simulink library "inp"  (R2021b)
settings: Solver=VariableStepAuto  StartTime=0.0  StopTime=10.0  RelTol=1e-3
undefined symbols (not defined in the file): C_TASK_5MS_S, FALSE, KINP_AcoreReadyToSlp_flg_ovrdflg, KINP_AcoreReadyToSlp_flg_ovrdval, KINP_AllowMovThd_OTA_enum_ovrdflg, KINP_AllowMovThd_OTA_enum_ovrdval, KINP_APSAngleTarget_Deg_ovrdflg, KINP_APSAngleTarget_Deg_ovrdval, KINP_APSDecReq_mps2_ovrdflg, KINP_APSDecReq_mps2_ovrdval, KINP_APSDecReqA_flg_ovrdflg, KINP_APSDecReqA_flg_ovrdval, KINP_APSDFLL_cm_ovrdflg, KINP_APSDFLL_cm_ovrdval, KINP_APSDFLR_cm_ovrdflg, KINP_APSDFLR_cm_ovrdval, KINP_APSDRLL_cm_ovrdflg, KINP_APSDRLL_cm_ovrdval, KINP_APSDRLR_cm_ovrdflg, KINP_APSDRLR_cm_ovrdval, KINP_APSExitCondition_enum_ovrdflg, KINP_APSExitCondition_enum_ovrdval, KINP_APSHWVer_enum_ovrdflg, KINP_APSHWVer_enum_ovrdval, KINP_APSProgressPCT_pct_ovrdflg, KINP_APSProgressPCT_pct_ovrdval, KINP_APSPwrReq_enum_ovrdflg, KINP_APSPwrReq_enum_ovrdval, KINP_APSReq_enum_ovrdflg, KINP_APSReq_enum_ovrdval, KINP_APSRQDisplay_enum_ovrdflg, KINP_APSRQDisplay_enum_ovrdval, KINP_APSRqEPASCtrl_flg_ovrdflg, KINP_APSRqEPASCtrl_flg_ovrdval, KINP_APSShiftPosnReq_enum_ovrdval, KINP_APSShiftPosnReq_enum_ovrflg, KINP_APSSpeedCMD_kph_ovrdval, KINP_APSSpeedCMD_kph_ovrflg, KINP_APSStaSystem_enum_ovrdflg, KINP_APSStaSystem_enum_ovrdval, KINP_APSSWVer_enum_ovrdflg, KINP_APSSWVer_enum_ovrdval, KINP_APSVMCReqA_flg_ovrdval, KINP_APSVMCReqA_flg_ovrflg, KINP_APSVRqEPASCtrl_flg_ovrdflg, KINP_APSVRqEPASCtrl_flg_ovrdval, KINP_AuxBattVolmV_mV_ovrdflg, KINP_AuxBattVolmV_mV_ovrdval, KINP_BTConnectSta_enum_ovrdflg, KINP_BTConnectSta_enum_ovrdval, KINP_CAASSta_enum_ovrdflg, KINP_CAASSta_enum_ovrdval, KINP_CAASVMCReqA_flg_ovrdval, KINP_CAASVMCReqA_flg_ovrflg, KINP_CAN1BusOff_flg_ovrdflg, KINP_CAN1BusOff_flg_ovrdval, KINP_CAN2BusOff_flg_ovrdflg, KINP_CAN2BusOff_flg_ovrdval, KINP_CAN3BusOff_flg_ovrdflg, KINP_CAN3BusOff_flg_ovrdval ... (+222)
libraries: FVT_lib x1035, hcu_lib x1
(part 30 of 33)

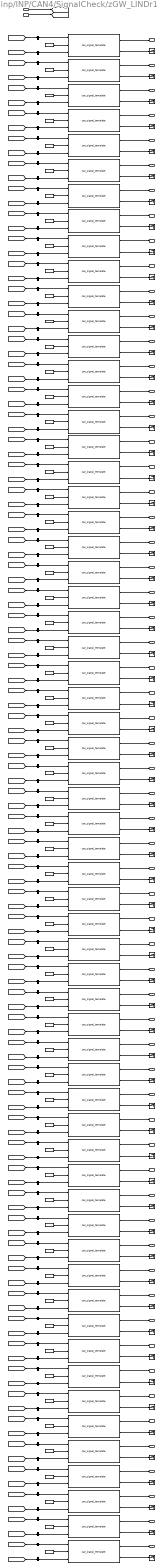
== system inp/INP/CAN4/SignalCheck/zGW_LINDr1 ==
  BHAL_outputs : Inport
  inp_CanValid_bus : Inport  Port=2
  CSWDimSw : FVT_lib/inp/can_signal_template  SystemSampleTime=-1  VariantActivationTime=update diagram  Latency=0  AutoFrameSizeCalculation=off
      link override defval: Value=KINP_CSWDimSw_flg_defval
      link override ovrdflg: Value=KINP_CSWDimSw_flg_ovrdflg
      link override ovrdval: Value=KINP_CSWDimSw_flg_ovrdval
  CSWFWasSwSta : FVT_lib/inp/can_signal_template  SystemSampleTime=-1  VariantActivationTime=update diagram  Latency=0  AutoFrameSizeCalculation=off
      link override defval: Value=KINP_CSWFWasSwSta_enum_defval
      link override ovrdflg: Value=KINP_CSWFWasSwSta_enum_ovrdflg
      link override ovrdval: Value=KINP_CSWFWasSwSta_enum_ovrdval
  CSWFWipSwSta : FVT_lib/inp/can_signal_template  SystemSampleTime=-1  VariantActivationTime=update diagram  Latency=0  AutoFrameSizeCalculation=off
      link override defval: Value=KINP_CSWFWipSwSta_enum_defval
      link override ovrdflg: Value=KINP_CSWFWipSwSta_enum_ovrdflg
      link override ovrdval: Value=KINP_CSWFWipSwSta_enum_ovrdval
  CSWPassSWSta : FVT_lib/inp/can_signal_template  SystemSampleTime=-1  VariantActivationTime=update diagram  Latency=0  AutoFrameSizeCalculation=off
      link override defval: Value=KINP_CSWPassSWSta_flg_defval
      link override ovrdflg: Value=KINP_CSWPassSWSta_flg_ovrdflg
      link override ovrdval: Value=KINP_CSWPassSWSta_flg_ovrdval
  CSWRWasSWSta : FVT_lib/inp/can_signal_template  SystemSampleTime=-1  VariantActivationTime=update diagram  Latency=0  AutoFrameSizeCalculation=off
      link override defval: Value=KINP_CSWRWasSWSta_enum_defval
      link override ovrdflg: Value=KINP_CSWRWasSWSta_enum_ovrdflg
      link override ovrdval: Value=KINP_CSWRWasSWSta_enum_ovrdval
  CSWRWipIntSwSta : FVT_lib/inp/can_signal_template  SystemSampleTime=-1  VariantActivationTime=update diagram  Latency=0  AutoFrameSizeCalculation=off
      link override defval: Value=KINP_CSWRWipIntSwSta_enum_defval
      link override ovrdflg: Value=KINP_CSWRWipIntSwSta_enum_ovrdflg
      link override ovrdval: Value=KINP_CSWRWipIntSwSta_enum_ovrdval
  CSWTurnSwSta : FVT_lib/inp/can_signal_template  SystemSampleTime=-1  VariantActivationTime=update diagram  Latency=0  AutoFrameSizeCalculation=off
      link override defval: Value=KINP_CSWTurnSwSta_enum_defval
      link override ovrdflg: Value=KINP_CSWTurnSwSta_enum_ovrdflg
      link override ovrdval: Value=KINP_CSWTurnSwSta_enum_ovrdval
  FAPWL01LINResponseError : FVT_lib/inp/can_signal_template  SystemSampleTime=-1  VariantActivationTime=update diagram  Latency=0  AutoFrameSizeCalculation=off
      link override defval: Value=KINP_FAPWL01LINResponseError_flg_defval
      link override ovrdflg: Value=KINP_FAPWL01LINResponseError_flg_ovrdflg
      link override ovrdval: Value=KINP_FAPWL01LINResponseError_flg_ovrdval
  LDrvMotorRelayError : FVT_lib/inp/can_signal_template  SystemSampleTime=-1  VariantActivationTime=update diagram  Latency=0  AutoFrameSizeCalculation=off
      link override defval: Value=KINP_LDrvMotorRelayError_flg_defval
      link override ovrdflg: Value=KINP_LDrvMotorRelayError_flg_ovrdflg
      link override ovrdval: Value=KINP_LDrvMotorRelayError_flg_ovrdval
  LDrvMotorRippleError : FVT_lib/inp/can_signal_template  SystemSampleTime=-1  VariantActivationTime=update diagram  Latency=0  AutoFrameSizeCalculation=off
      link override defval: Value=KINP_LDrvMotorRippleError_flg_defval
      link override ovrdflg: Value=KINP_LDrvMotorRippleError_flg_ovrdflg
      link override ovrdval: Value=KINP_LDrvMotorRippleError_flg_ovrdval
  LDrvValWdwOpened : FVT_lib/inp/can_signal_template  SystemSampleTime=-1  VariantActivationTime=update diagram  Latency=0  AutoFrameSizeCalculation=off
      link override defval: Value=KINP_LDrvValWdwOpened_pct_defval
      link override ovrdflg: Value=KINP_LDrvValWdwOpened_pct_ovrdflg
      link override ovrdval: Value=KINP_LDrvValWdwOpened_pct_ovrdval
  LDrvWdwPositionSts : FVT_lib/inp/can_signal_template  SystemSampleTime=-1  VariantActivationTime=update diagram  Latency=0  AutoFrameSizeCalculation=off
      link override defval: Value=KINP_LDrvWdwPositionSts_enum_defval
      link override ovrdflg: Value=KINP_LDrvWdwPositionSts_enum_ovrdflg
      link override ovrdval: Value=KINP_LDrvWdwPositionSts_enum_ovrdval
  LPasMotorRelayError : FVT_lib/inp/can_signal_template  SystemSampleTime=-1  VariantActivationTime=update diagram  Latency=0  AutoFrameSizeCalculation=off
      link override defval: Value=KINP_LPasMotorRelayError_flg_defval
      link override ovrdflg: Value=KINP_LPasMotorRelayError_flg_ovrdflg
      link override ovrdval: Value=KINP_LPasMotorRelayError_flg_ovrdval
  LPasMotorRippleError : FVT_lib/inp/can_signal_template  SystemSampleTime=-1  VariantActivationTime=update diagram  Latency=0  AutoFrameSizeCalculation=off
      link override defval: Value=KINP_LPasMotorRippleError_flg_defval
      link override ovrdflg: Value=KINP_LPasMotorRippleError_flg_ovrdflg
      link override ovrdval: Value=KINP_LPasMotorRippleError_flg_ovrdval
  LPasValWdwOpened : FVT_lib/inp/can_signal_template  SystemSampleTime=-1  VariantActivationTime=update diagram  Latency=0  AutoFrameSizeCalculation=off
      link override defval: Value=KINP_LPasValWdwOpened_pct_defval
      link override ovrdflg: Value=KINP_LPasValWdwOpened_pct_ovrdflg
      link override ovrdval: Value=KINP_LPasValWdwOpened_pct_ovrdval
  LPasWdwPositionSts : FVT_lib/inp/can_signal_template  SystemSampleTime=-1  VariantActivationTime=update diagram  Latency=0  AutoFrameSizeCalculation=off
      link override defval: Value=KINP_LPasWdwPositionSts_enum_defval
      link override ovrdflg: Value=KINP_LPasWdwPositionSts_enum_ovrdflg
      link override ovrdval: Value=KINP_LPasWdwPositionSts_enum_ovrdval
  LRLDMotorRelayError : FVT_lib/inp/can_signal_template  SystemSampleTime=-1  VariantActivationTime=update diagram  Latency=0  AutoFrameSizeCalculation=off
      link override defval: Value=KINP_LRLDMotorRelayError_flg_defval
      link override ovrdflg: Value=KINP_LRLDMotorRelayError_flg_ovrdflg
      link override ovrdval: Value=KINP_LRLDMotorRelayError_flg_ovrdval
  LRLDMotorRippleError : FVT_lib/inp/can_signal_template  SystemSampleTime=-1  VariantActivationTime=update diagram  Latency=0  AutoFrameSizeCalculation=off
      link override defval: Value=KINP_LRLDMotorRippleError_flg_defval
      link override ovrdflg: Value=KINP_LRLDMotorRippleError_flg_ovrdflg
      link override ovrdval: Value=KINP_LRLDMotorRippleError_flg_ovrdval
  LRLDValWdwOpened : FVT_lib/inp/can_signal_template  SystemSampleTime=-1  VariantActivationTime=update diagram  Latency=0  AutoFrameSizeCalculation=off
      link override defval: Value=KINP_LRLDValWdwOpened_pct_defval
      link override ovrdflg: Value=KINP_LRLDValWdwOpened_pct_ovrdflg
      link override ovrdval: Value=KINP_LRLDValWdwOpened_pct_ovrdval
  LRLDWdwPositionSts : FVT_lib/inp/can_signal_template  SystemSampleTime=-1  VariantActivationTime=update diagram  Latency=0  AutoFrameSizeCalculation=off
      link override defval: Value=KINP_LRLDWdwPositionSts_enum_defval
      link override ovrdflg: Value=KINP_LRLDWdwPositionSts_enum_ovrdflg
      link override ovrdval: Value=KINP_LRLDWdwPositionSts_enum_ovrdval
  LRRDMotorRelayError : FVT_lib/inp/can_signal_template  SystemSampleTime=-1  VariantActivationTime=update diagram  Latency=0  AutoFrameSizeCalculation=off
      link override defval: Value=KINP_LRRDMotorRelayError_flg_defval
      link override ovrdflg: Value=KINP_LRRDMotorRelayError_flg_ovrdflg
      link override ovrdval: Value=KINP_LRRDMotorRelayError_flg_ovrdval
  LRRDMotorRippleError : FVT_lib/inp/can_signal_template  SystemSampleTime=-1  VariantActivationTime=update diagram  Latency=0  AutoFrameSizeCalculation=off
      link override defval: Value=KINP_LRRDMotorRippleError_flg_defval
      link override ovrdflg: Value=KINP_LRRDMotorRippleError_flg_ovrdflg
      link override ovrdval: Value=KINP_LRRDMotorRippleError_flg_ovrdval
  LRRDValWdwOpened : FVT_lib/inp/can_signal_template  SystemSampleTime=-1  VariantActivationTime=update diagram  Latency=0  AutoFrameSizeCalculation=off
      link override defval: Value=KINP_LRRDValWdwOpened_pct_defval
      link override ovrdflg: Value=KINP_LRRDValWdwOpened_pct_ovrdflg
      link override ovrdval: Value=KINP_LRRDValWdwOpened_pct_ovrdval
  LRRDWdwPositionSts : FVT_lib/inp/can_signal_template  SystemSampleTime=-1  VariantActivationTime=update diagram  Latency=0  AutoFrameSizeCalculation=off
      link override defval: Value=KINP_LRRDWdwPositionSts_enum_defval
      link override ovrdflg: Value=KINP_LRRDWdwPositionSts_enum_ovrdflg
      link override ovrdval: Value=KINP_LRRDWdwPositionSts_enum_ovrdval
  RAPWL01LINResponseError : FVT_lib/inp/can_signal_template  SystemSampleTime=-1  VariantActivationTime=update diagram  Latency=0  AutoFrameSizeCalculation=off
      link override defval: Value=KINP_RAPWL01LINResponseError_flg_defval
      link override ovrdflg: Value=KINP_RAPWL01LINResponseError_flg_ovrdflg
      link override ovrdval: Value=KINP_RAPWL01LINResponseError_flg_ovrdval
  RLSLampSta : FVT_lib/inp/can_signal_template  SystemSampleTime=-1  VariantActivationTime=update diagram  Latency=0  AutoFrameSizeCalculation=off
      link override defval: Value=KINP_RLSLampSta_flg_defval
      link override ovrdflg: Value=KINP_RLSLampSta_flg_ovrdflg
      link override ovrdval: Value=KINP_RLSLampSta_flg_ovrdval
  RLSRainSnrWiperCmd : FVT_lib/inp/can_signal_template  SystemSampleTime=-1  VariantActivationTime=update diagram  Latency=0  AutoFrameSizeCalculation=off
      link override defval: Value=KINP_RLSRainSnrWiperCmd_enum_defval
      link override ovrdflg: Value=KINP_RLSRainSnrWiperCmd_enum_ovrdflg
      link override ovrdval: Value=KINP_RLSRainSnrWiperCmd_enum_ovrdval
  SWC2LADASSta : FVT_lib/inp/can_signal_template  SystemSampleTime=-1  VariantActivationTime=update diagram  Latency=0  AutoFrameSizeCalculation=off
      link override defval: Value=KINP_SWC2LADASSta_flg_defval
      link override ovrdflg: Value=KINP_SWC2LADASSta_flg_ovrdflg
      link override ovrdval: Value=KINP_SWC2LADASSta_flg_ovrdval
  SWC2LDriveModeSta : FVT_lib/inp/can_signal_template  SystemSampleTime=-1  VariantActivationTime=update diagram  Latency=0  AutoFrameSizeCalculation=off
      link override defval: Value=KINP_SWC2LDriveModeSta_flg_defval
      link override ovrdflg: Value=KINP_SWC2LDriveModeSta_flg_ovrdflg
      link override ovrdval: Value=KINP_SWC2LDriveModeSta_flg_ovrdval
  SWC2LHomeSta : FVT_lib/inp/can_signal_template  SystemSampleTime=-1  VariantActivationTime=update diagram  Latency=0  AutoFrameSizeCalculation=off
      link override defval: Value=KINP_SWC2LHomeSta_flg_defval
      link override ovrdflg: Value=KINP_SWC2LHomeSta_flg_ovrdflg
      link override ovrdval: Value=KINP_SWC2LHomeSta_flg_ovrdval
  SWC2LLeftSta : FVT_lib/inp/can_signal_template  SystemSampleTime=-1  VariantActivationTime=update diagram  Latency=0  AutoFrameSizeCalculation=off
      link override defval: Value=KINP_SWC2LLeftSta_flg_defval
      link override ovrdflg: Value=KINP_SWC2LLeftSta_flg_ovrdflg
      link override ovrdval: Value=KINP_SWC2LLeftSta_flg_ovrdval
  SWC2LRegenUpSta : FVT_lib/inp/can_signal_template  SystemSampleTime=-1  VariantActivationTime=update diagram  Latency=0  AutoFrameSizeCalculation=off
      link override defval: Value=KINP_SWC2LRegenUpSta_flg_defval
      link override ovrdflg: Value=KINP_SWC2LRegenUpSta_flg_ovrdflg
      link override ovrdval: Value=KINP_SWC2LRegenUpSta_flg_ovrdval
  SWC2LRightSta : FVT_lib/inp/can_signal_template  SystemSampleTime=-1  VariantActivationTime=update diagram  Latency=0  AutoFrameSizeCalculation=off
      link override defval: Value=KINP_SWC2LRightSta_flg_defval
      link override ovrdflg: Value=KINP_SWC2LRightSta_flg_ovrdflg
      link override ovrdval: Value=KINP_SWC2LRightSta_flg_ovrdval
  SWC2LScrollDownSta : FVT_lib/inp/can_signal_template  SystemSampleTime=-1  VariantActivationTime=update diagram  Latency=0  AutoFrameSizeCalculation=off
      link override defval: Value=KINP_SWC2LScrollDownSta_flg_defval
      link override ovrdflg: Value=KINP_SWC2LScrollDownSta_flg_ovrdflg
      link override ovrdval: Value=KINP_SWC2LScrollDownSta_flg_ovrdval
  SWC2LScrollPressSta : FVT_lib/inp/can_signal_template  SystemSampleTime=-1  VariantActivationTime=update diagram  Latency=0  AutoFrameSizeCalculation=off
      link override defval: Value=KINP_SWC2LScrollPressSta_flg_defval
      link override ovrdflg: Value=KINP_SWC2LScrollPressSta_flg_ovrdflg
      link override ovrdval: Value=KINP_SWC2LScrollPressSta_flg_ovrdval
  SWC2LScrollUpSta : FVT_lib/inp/can_signal_template  SystemSampleTime=-1  VariantActivationTime=update diagram  Latency=0  AutoFrameSizeCalculation=off
      link override defval: Value=KINP_SWC2LScrollUpSta_flg_defval
      link override ovrdflg: Value=KINP_SWC2LScrollUpSta_flg_ovrdflg
      link override ovrdval: Value=KINP_SWC2LScrollUpSta_flg_ovrdval
  SWC2RCustomizeSta : FVT_lib/inp/can_signal_template  SystemSampleTime=-1  VariantActivationTime=update diagram  Latency=0  AutoFrameSizeCalculation=off
      link override defval: Value=KINP_SWC2RCustomizeSta_flg_defval
      link override ovrdflg: Value=KINP_SWC2RCustomizeSta_flg_ovrdflg
      link override ovrdval: Value=KINP_SWC2RCustomizeSta_flg_ovrdval
  SWC2RLeftSta : FVT_lib/inp/can_signal_template  SystemSampleTime=-1  VariantActivationTime=update diagram  Latency=0  AutoFrameSizeCalculation=off
      link override defval: Value=KINP_SWC2RLeftSta_flg_defval
      link override ovrdflg: Value=KINP_SWC2RLeftSta_flg_ovrdflg
      link override ovrdval: Value=KINP_SWC2RLeftSta_flg_ovrdval
  SWC2RPageSwitchSta : FVT_lib/inp/can_signal_template  SystemSampleTime=-1  VariantActivationTime=update diagram  Latency=0  AutoFrameSizeCalculation=off
      link override defval: Value=KINP_SWC2RPageSwitchSta_flg_defval
      link override ovrdflg: Value=KINP_SWC2RPageSwitchSta_flg_ovrdflg
      link override ovrdval: Value=KINP_SWC2RPageSwitchSta_flg_ovrdval
  SWC2RRegenDownSta : FVT_lib/inp/can_signal_template  SystemSampleTime=-1  VariantActivationTime=update diagram  Latency=0  AutoFrameSizeCalculation=off
      link override defval: Value=KINP_SWC2RRegenDownSta_flg_defval
      link override ovrdflg: Value=KINP_SWC2RRegenDownSta_flg_ovrdflg
      link override ovrdval: Value=KINP_SWC2RRegenDownSta_flg_ovrdval
  SWC2RRightSta : FVT_lib/inp/can_signal_template  SystemSampleTime=-1  VariantActivationTime=update diagram  Latency=0  AutoFrameSizeCalculation=off
      link override defval: Value=KINP_SWC2RRightSta_flg_defval
      link override ovrdflg: Value=KINP_SWC2RRightSta_flg_ovrdflg
      link override ovrdval: Value=KINP_SWC2RRightSta_flg_ovrdval
  SWC2RScrollDownSta : FVT_lib/inp/can_signal_template  SystemSampleTime=-1  VariantActivationTime=update diagram  Latency=0  AutoFrameSizeCalculation=off
      link override defval: Value=KINP_SWC2RScrollDownSta_flg_defval
      link override ovrdflg: Value=KINP_SWC2RScrollDownSta_flg_ovrdflg
      link override ovrdval: Value=KINP_SWC2RScrollDownSta_flg_ovrdval
  SWC2RScrollPressSta : FVT_lib/inp/can_signal_template  SystemSampleTime=-1  VariantActivationTime=update diagram  Latency=0  AutoFrameSizeCalculation=off
      link override defval: Value=KINP_SWC2RScrollPressSta_flg_defval
      link override ovrdflg: Value=KINP_SWC2RScrollPressSta_flg_ovrdflg
      link override ovrdval: Value=KINP_SWC2RScrollPressSta_flg_ovrdval
  SWC2RScrollUpSta : FVT_lib/inp/can_signal_template  SystemSampleTime=-1  VariantActivationTime=update diagram  Latency=0  AutoFrameSizeCalculation=off
      link override defval: Value=KINP_SWC2RScrollUpSta_flg_defval
      link override ovrdflg: Value=KINP_SWC2RScrollUpSta_flg_ovrdflg
      link override ovrdval: Value=KINP_SWC2RScrollUpSta_flg_ovrdval
  SWC2RVRSta : FVT_lib/inp/can_signal_template  SystemSampleTime=-1  VariantActivationTime=update diagram  Latency=0  AutoFrameSizeCalculation=off
      link override defval: Value=KINP_SWC2RVRSta_flg_defval
      link override ovrdflg: Value=KINP_SWC2RVRSta_flg_ovrdflg
      link override ovrdval: Value=KINP_SWC2RVRSta_flg_ovrdval
  SWCACCSta : FVT_lib/inp/can_signal_template  SystemSampleTime=-1  VariantActivationTime=update diagram  Latency=0  AutoFrameSizeCalculation=off
      link override defval: Value=KINP_SWCACCSta_flg_defval
      link override ovrdflg: Value=KINP_SWCACCSta_flg_ovrdflg
      link override ovrdval: Value=KINP_SWCACCSta_flg_ovrdval
  SWCCANCELSta : FVT_lib/inp/can_signal_template  SystemSampleTime=-1  VariantActivationTime=update diagram  Latency=0  AutoFrameSizeCalculation=off
      link override defval: Value=KINP_SWCCANCELSta_flg_defval
      link override ovrdflg: Value=KINP_SWCCANCELSta_flg_ovrdflg
      link override ovrdval: Value=KINP_SWCCANCELSta_flg_ovrdval
  SWCDistanceSta : FVT_lib/inp/can_signal_template  SystemSampleTime=-1  VariantActivationTime=update diagram  Latency=0  AutoFrameSizeCalculation=off
      link override defval: Value=KINP_SWCDistanceSta_flg_defval
      link override ovrdflg: Value=KINP_SWCDistanceSta_flg_ovrdflg
      link override ovrdval: Value=KINP_SWCDistanceSta_flg_ovrdval
  SWCDownSta : FVT_lib/inp/can_signal_template  SystemSampleTime=-1  VariantActivationTime=update diagram  Latency=0  AutoFrameSizeCalculation=off
      link override defval: Value=KINP_SWCDownSta_flg_defval
      link override ovrdflg: Value=KINP_SWCDownSta_flg_ovrdflg
      link override ovrdval: Value=KINP_SWCDownSta_flg_ovrdval
  SWCLKASta : FVT_lib/inp/can_signal_template  SystemSampleTime=-1  VariantActivationTime=update diagram  Latency=0  AutoFrameSizeCalculation=off
      link override defval: Value=KINP_SWCLKASta_flg_defval
      link override ovrdflg: Value=KINP_SWCLKASta_flg_ovrdflg
      link override ovrdval: Value=KINP_SWCLKASta_flg_ovrdval
  SWCLeftSta : FVT_lib/inp/can_signal_template  SystemSampleTime=-1  VariantActivationTime=update diagram  Latency=0  AutoFrameSizeCalculation=off
      link override defval: Value=KINP_SWCLeftSta_flg_defval
      link override ovrdflg: Value=KINP_SWCLeftSta_flg_ovrdflg
      link override ovrdval: Value=KINP_SWCLeftSta_flg_ovrdval
  SWCRegenDown : FVT_lib/inp/can_signal_template  SystemSampleTime=-1  VariantActivationTime=update diagram  Latency=0  AutoFrameSizeCalculation=off
      link override defval: Value=KINP_SWCRegenDown_flg_defval
      link override ovrdflg: Value=KINP_SWCRegenDown_flg_ovrdflg
      link override ovrdval: Value=KINP_SWCRegenDown_flg_ovrdval
  SWCRegenUp : FVT_lib/inp/can_signal_template  SystemSampleTime=-1  VariantActivationTime=update diagram  Latency=0  AutoFrameSizeCalculation=off
      link override defval: Value=KINP_SWCRegenUp_flg_defval
      link override ovrdflg: Value=KINP_SWCRegenUp_flg_ovrdflg
      link override ovrdval: Value=KINP_SWCRegenUp_flg_ovrdval
  SWCResUpSta : FVT_lib/inp/can_signal_template  SystemSampleTime=-1  VariantActivationTime=update diagram  Latency=0  AutoFrameSizeCalculation=off
      link override defval: Value=KINP_SWCResUpSta_flg_defval
      link override ovrdflg: Value=KINP_SWCResUpSta_flg_ovrdflg
      link override ovrdval: Value=KINP_SWCResUpSta_flg_ovrdval
  SWCRightSta : FVT_lib/inp/can_signal_template  SystemSampleTime=-1  VariantActivationTime=update diagram  Latency=0  AutoFrameSizeCalculation=off
      link override defval: Value=KINP_SWCRightSta_flg_defval
      link override ovrdflg: Value=KINP_SWCRightSta_flg_ovrdflg
      link override ovrdval: Value=KINP_SWCRightSta_flg_ovrdval
  SWCSetdownSta : FVT_lib/inp/can_signal_template  SystemSampleTime=-1  VariantActivationTime=update diagram  Latency=0  AutoFrameSizeCalculation=off
      link override defval: Value=KINP_SWCSetdownSta_flg_defval
      link override ovrdflg: Value=KINP_SWCSetdownSta_flg_ovrdflg
      link override ovrdval: Value=KINP_SWCSetdownSta_flg_ovrdval
  SWCTripSta : FVT_lib/inp/can_signal_template  SystemSampleTime=-1  VariantActivationTime=update diagram  Latency=0  AutoFrameSizeCalculation=off
      link override defval: Value=KINP_SWCTripSta_flg_defval
      link override ovrdflg: Value=KINP_SWCTripSta_flg_ovrdflg
      link override ovrdval: Value=KINP_SWCTripSta_flg_ovrdval
  SWCUndefinedSta : FVT_lib/inp/can_signal_template  SystemSampleTime=-1  VariantActivationTime=update diagram  Latency=0  AutoFrameSizeCalculation=off
      link override defval: Value=KINP_SWCUndefinedSta_flg_defval
      link override ovrdflg: Value=KINP_SWCUndefinedSta_flg_ovrdflg
      link override ovrdval: Value=KINP_SWCUndefinedSta_flg_ovrdval
  SWCUpSta : FVT_lib/inp/can_signal_template  SystemSampleTime=-1  VariantActivationTime=update diagram  Latency=0  AutoFrameSizeCalculation=off
      link override defval: Value=KINP_SWCUpSta_flg_defval
      link override ovrdflg: Value=KINP_SWCUpSta_flg_ovrdflg
      link override ovrdval: Value=KINP_SWCUpSta_flg_ovrdval
  SWCVRSta : FVT_lib/inp/can_signal_template  SystemSampleTime=-1  VariantActivationTime=update diagram  Latency=0  AutoFrameSizeCalculation=off
      link override defval: Value=KINP_SWCVRSta_flg_defval
      link override ovrdflg: Value=KINP_SWCVRSta_flg_ovrdflg
      link override ovrdval: Value=KINP_SWCVRSta_flg_ovrdval
  SWCmodeSta : FVT_lib/inp/can_signal_template  SystemSampleTime=-1  VariantActivationTime=update diagram  Latency=0  AutoFrameSizeCalculation=off
      link override defval: Value=KINP_SWCmodeSta_flg_defval
      link override ovrdflg: Value=KINP_SWCmodeSta_flg_ovrdflg
      link override ovrdval: Value=KINP_SWCmodeSta_flg_ovrdval
  Terminator_{1..61} (61 alike) : Terminator
  True_VHAL_CSWDimSw_flg : Constant  Value=TRUE  OutDataTypeStr=boolean
  True_VHAL_CSWFWasSwSta_enum : Constant  Value=TRUE  OutDataTypeStr=boolean
  True_VHAL_CSWFWipSwSta_enum : Constant  Value=TRUE  OutDataTypeStr=boolean
  True_VHAL_CSWPassSWSta_flg : Constant  Value=TRUE  OutDataTypeStr=boolean
  True_VHAL_CSWRWasSWSta_enum : Constant  Value=TRUE  OutDataTypeStr=boolean
  True_VHAL_CSWRWipIntSwSta_enum : Constant  Value=TRUE  OutDataTypeStr=boolean
  True_VHAL_CSWTurnSwSta_enum : Constant  Value=TRUE  OutDataTypeStr=boolean
  True_VHAL_FAPWL01LINResponseError_flg : Constant  Value=TRUE  OutDataTypeStr=boolean
  True_VHAL_LDrvMotorRelayError_flg : Constant  Value=TRUE  OutDataTypeStr=boolean
  True_VHAL_LDrvMotorRippleError_flg : Constant  Value=TRUE  OutDataTypeStr=boolean
  True_VHAL_LDrvValWdwOpened_pct : Constant  Value=TRUE  OutDataTypeStr=boolean
  True_VHAL_LDrvWdwPositionSts_enum : Constant  Value=TRUE  OutDataTypeStr=boolean
  True_VHAL_LPasMotorRelayError_flg : Constant  Value=TRUE  OutDataTypeStr=boolean
  True_VHAL_LPasMotorRippleError_flg : Constant  Value=TRUE  OutDataTypeStr=boolean
  True_VHAL_LPasValWdwOpened_pct : Constant  Value=TRUE  OutDataTypeStr=boolean
  True_VHAL_LPasWdwPositionSts_enum : Constant  Value=TRUE  OutDataTypeStr=boolean
  True_VHAL_LRLDMotorRelayError_flg : Constant  Value=TRUE  OutDataTypeStr=boolean
  True_VHAL_LRLDMotorRippleError_flg : Constant  Value=TRUE  OutDataTypeStr=boolean
  True_VHAL_LRLDValWdwOpened_pct : Constant  Value=TRUE  OutDataTypeStr=boolean
  True_VHAL_LRLDWdwPositionSts_enum : Constant  Value=TRUE  OutDataTypeStr=boolean
  True_VHAL_LRRDMotorRelayError_flg : Constant  Value=TRUE  OutDataTypeStr=boolean
  True_VHAL_LRRDMotorRippleError_flg : Constant  Value=TRUE  OutDataTypeStr=boolean
  True_VHAL_LRRDValWdwOpened_pct : Constant  Value=TRUE  OutDataTypeStr=boolean
  True_VHAL_LRRDWdwPositionSts_enum : Constant  Value=TRUE  OutDataTypeStr=boolean
  True_VHAL_RAPWL01LINResponseError_flg : Constant  Value=TRUE  OutDataTypeStr=boolean
  True_VHAL_RLSLampSta_flg : Constant  Value=TRUE  OutDataTypeStr=boolean
  True_VHAL_RLSRainSnrWiperCmd_enum : Constant  Value=TRUE  OutDataTypeStr=boolean
  True_VHAL_SWC2LADASSta_flg : Constant  Value=TRUE  OutDataTypeStr=boolean
  True_VHAL_SWC2LDriveModeSta_flg : Constant  Value=TRUE  OutDataTypeStr=boolean
  True_VHAL_SWC2LHomeSta_flg : Constant  Value=TRUE  OutDataTypeStr=boolean
  True_VHAL_SWC2LLeftSta_flg : Constant  Value=TRUE  OutDataTypeStr=boolean
  True_VHAL_SWC2LRegenUpSta_flg : Constant  Value=TRUE  OutDataTypeStr=boolean
  True_VHAL_SWC2LRightSta_flg : Constant  Value=TRUE  OutDataTypeStr=boolean
  True_VHAL_SWC2LScrollDownSta_flg : Constant  Value=TRUE  OutDataTypeStr=boolean
  True_VHAL_SWC2LScrollPressSta_flg : Constant  Value=TRUE  OutDataTypeStr=boolean
  True_VHAL_SWC2LScrollUpSta_flg : Constant  Value=TRUE  OutDataTypeStr=boolean
  True_VHAL_SWC2RCustomizeSta_flg : Constant  Value=TRUE  OutDataTypeStr=boolean
  True_VHAL_SWC2RLeftSta_flg : Constant  Value=TRUE  OutDataTypeStr=boolean
  True_VHAL_SWC2RPageSwitchSta_flg : Constant  Value=TRUE  OutDataTypeStr=boolean
  True_VHAL_SWC2RRegenDownSta_flg : Constant  Value=TRUE  OutDataTypeStr=boolean
  True_VHAL_SWC2RRightSta_flg : Constant  Value=TRUE  OutDataTypeStr=boolean
  True_VHAL_SWC2RScrollDownSta_flg : Constant  Value=TRUE  OutDataTypeStr=boolean
  True_VHAL_SWC2RScrollPressSta_flg : Constant  Value=TRUE  OutDataTypeStr=boolean
  True_VHAL_SWC2RScrollUpSta_flg : Constant  Value=TRUE  OutDataTypeStr=boolean
  True_VHAL_SWC2RVRSta_flg : Constant  Value=TRUE  OutDataTypeStr=boolean
  True_VHAL_SWCACCSta_flg : Constant  Value=TRUE  OutDataTypeStr=boolean
  True_VHAL_SWCCANCELSta_flg : Constant  Value=TRUE  OutDataTypeStr=boolean
  True_VHAL_SWCDistanceSta_flg : Constant  Value=TRUE  OutDataTypeStr=boolean
  True_VHAL_SWCDownSta_flg : Constant  Value=TRUE  OutDataTypeStr=boolean
  True_VHAL_SWCLKASta_flg : Constant  Value=TRUE  OutDataTypeStr=boolean
  True_VHAL_SWCLeftSta_flg : Constant  Value=TRUE  OutDataTypeStr=boolean
  True_VHAL_SWCRegenDown_flg : Constant  Value=TRUE  OutDataTypeStr=boolean
  True_VHAL_SWCRegenUp_flg : Constant  Value=TRUE  OutDataTypeStr=boolean
  True_VHAL_SWCResUpSta_flg : Constant  Value=TRUE  OutDataTypeStr=boolean
  True_VHAL_SWCRightSta_flg : Constant  Value=TRUE  OutDataTypeStr=boolean
  True_VHAL_SWCSetdownSta_flg : Constant  Value=TRUE  OutDataTypeStr=boolean
  True_VHAL_SWCTripSta_flg : Constant  Value=TRUE  OutDataTypeStr=boolean
  True_VHAL_SWCUndefinedSta_flg : Constant  Value=TRUE  OutDataTypeStr=boolean
  True_VHAL_SWCUpSta_flg : Constant  Value=TRUE  OutDataTypeStr=boolean
  True_VHAL_SWCVRSta_flg : Constant  Value=TRUE  OutDataTypeStr=boolean
  True_VHAL_SWCmodeSta_flg : Constant  Value=TRUE  OutDataTypeStr=boolean
  slr1_{1..61} (61 alike) : BusSelector  OutputSignals=VINP_CANMsgValidzGWLINDr1_flg
  slr_VHAL_CSWDimSw_flg : BusSelector  OutputSignals=VHAL_CSWDimSw_flg
  slr_VHAL_CSWFWasSwSta_enum : BusSelector  OutputSignals=VHAL_CSWFWasSwSta_enum
  slr_VHAL_CSWFWipSwSta_enum : BusSelector  OutputSignals=VHAL_CSWFWipSwSta_enum
  slr_VHAL_CSWPassSWSta_flg : BusSelector  OutputSignals=VHAL_CSWPassSWSta_flg
  slr_VHAL_CSWRWasSWSta_enum : BusSelector  OutputSignals=VHAL_CSWRWasSWSta_enum
  slr_VHAL_CSWRWipIntSwSta_enum : BusSelector  OutputSignals=VHAL_CSWRWipIntSwSta_enum
  slr_VHAL_CSWTurnSwSta_enum : BusSelector  OutputSignals=VHAL_CSWTurnSwSta_enum
  slr_VHAL_FAPWL01LINResponseError_flg : BusSelector  OutputSignals=VHAL_FAPWL01LINResponseError_flg
  slr_VHAL_LDrvMotorRelayError_flg : BusSelector  OutputSignals=VHAL_LDrvMotorRelayError_flg
  slr_VHAL_LDrvMotorRippleError_flg : BusSelector  OutputSignals=VHAL_LDrvMotorRippleError_flg
  slr_VHAL_LDrvValWdwOpened_pct : BusSelector  OutputSignals=VHAL_LDrvValWdwOpened_pct
  slr_VHAL_LDrvWdwPositionSts_enum : BusSelector  OutputSignals=VHAL_LDrvWdwPositionSts_enum
  slr_VHAL_LPasMotorRelayError_flg : BusSelector  OutputSignals=VHAL_LPasMotorRelayError_flg
  slr_VHAL_LPasMotorRippleError_flg : BusSelector  OutputSignals=VHAL_LPasMotorRippleError_flg
  slr_VHAL_LPasValWdwOpened_pct : BusSelector  OutputSignals=VHAL_LPasValWdwOpened_pct
  slr_VHAL_LPasWdwPositionSts_enum : BusSelector  OutputSignals=VHAL_LPasWdwPositionSts_enum
  slr_VHAL_LRLDMotorRelayError_flg : BusSelector  OutputSignals=VHAL_LRLDMotorRelayError_flg
  slr_VHAL_LRLDMotorRippleError_flg : BusSelector  OutputSignals=VHAL_LRLDMotorRippleError_flg
  slr_VHAL_LRLDValWdwOpened_pct : BusSelector  OutputSignals=VHAL_LRLDValWdwOpened_pct
  slr_VHAL_LRLDWdwPositionSts_enum : BusSelector  OutputSignals=VHAL_LRLDWdwPositionSts_enum
  slr_VHAL_LRRDMotorRelayError_flg : BusSelector  OutputSignals=VHAL_LRRDMotorRelayError_flg
  slr_VHAL_LRRDMotorRippleError_flg : BusSelector  OutputSignals=VHAL_LRRDMotorRippleError_flg
  slr_VHAL_LRRDValWdwOpened_pct : BusSelector  OutputSignals=VHAL_LRRDValWdwOpened_pct
  slr_VHAL_LRRDWdwPositionSts_enum : BusSelector  OutputSignals=VHAL_LRRDWdwPositionSts_enum
  slr_VHAL_RAPWL01LINResponseError_flg : BusSelector  OutputSignals=VHAL_RAPWL01LINResponseError_flg
  slr_VHAL_RLSLampSta_flg : BusSelector  OutputSignals=VHAL_RLSLampSta_flg
  slr_VHAL_RLSRainSnrWiperCmd_enum : BusSelector  OutputSignals=VHAL_RLSRainSnrWiperCmd_enum
  slr_VHAL_SWC2LADASSta_flg : BusSelector  OutputSignals=VHAL_SWC2LADASSta_flg
  slr_VHAL_SWC2LDriveModeSta_flg : BusSelector  OutputSignals=VHAL_SWC2LDriveModeSta_flg
  slr_VHAL_SWC2LHomeSta_flg : BusSelector  OutputSignals=VHAL_SWC2LHomeSta_flg
  slr_VHAL_SWC2LLeftSta_flg : BusSelector  OutputSignals=VHAL_SWC2LLeftSta_flg
  slr_VHAL_SWC2LRegenUpSta_flg : BusSelector  OutputSignals=VHAL_SWC2LRegenUpSta_flg
  slr_VHAL_SWC2LRightSta_flg : BusSelector  OutputSignals=VHAL_SWC2LRightSta_flg
  slr_VHAL_SWC2LScrollDownSta_flg : BusSelector  OutputSignals=VHAL_SWC2LScrollDownSta_flg
  slr_VHAL_SWC2LScrollPressSta_flg : BusSelector  OutputSignals=VHAL_SWC2LScrollPressSta_flg
  slr_VHAL_SWC2LScrollUpSta_flg : BusSelector  OutputSignals=VHAL_SWC2LScrollUpSta_flg
  slr_VHAL_SWC2RCustomizeSta_flg : BusSelector  OutputSignals=VHAL_SWC2RCustomizeSta_flg
  slr_VHAL_SWC2RLeftSta_flg : BusSelector  OutputSignals=VHAL_SWC2RLeftSta_flg
  slr_VHAL_SWC2RPageSwitchSta_flg : BusSelector  OutputSignals=VHAL_SWC2RPageSwitchSta_flg
  slr_VHAL_SWC2RRegenDownSta_flg : BusSelector  OutputSignals=VHAL_SWC2RRegenDownSta_flg
  slr_VHAL_SWC2RRightSta_flg : BusSelector  OutputSignals=VHAL_SWC2RRightSta_flg
  slr_VHAL_SWC2RScrollDownSta_flg : BusSelector  OutputSignals=VHAL_SWC2RScrollDownSta_flg
  slr_VHAL_SWC2RScrollPressSta_flg : BusSelector  OutputSignals=VHAL_SWC2RScrollPressSta_flg
  slr_VHAL_SWC2RScrollUpSta_flg : BusSelector  OutputSignals=VHAL_SWC2RScrollUpSta_flg
  slr_VHAL_SWC2RVRSta_flg : BusSelector  OutputSignals=VHAL_SWC2RVRSta_flg
  slr_VHAL_SWCACCSta_flg : BusSelector  OutputSignals=VHAL_SWCACCSta_flg
  slr_VHAL_SWCCANCELSta_flg : BusSelector  OutputSignals=VHAL_SWCCANCELSta_flg
  slr_VHAL_SWCDistanceSta_flg : BusSelector  OutputSignals=VHAL_SWCDistanceSta_flg
  slr_VHAL_SWCDownSta_flg : BusSelector  OutputSignals=VHAL_SWCDownSta_flg
  slr_VHAL_SWCLKASta_flg : BusSelector  OutputSignals=VHAL_SWCLKASta_flg
  slr_VHAL_SWCLeftSta_flg : BusSelector  OutputSignals=VHAL_SWCLeftSta_flg
  slr_VHAL_SWCRegenDown_flg : BusSelector  OutputSignals=VHAL_SWCRegenDown_flg
  slr_VHAL_SWCRegenUp_flg : BusSelector  OutputSignals=VHAL_SWCRegenUp_flg
  slr_VHAL_SWCResUpSta_flg : BusSelector  OutputSignals=VHAL_SWCResUpSta_flg
  slr_VHAL_SWCRightSta_flg : BusSelector  OutputSignals=VHAL_SWCRightSta_flg
  slr_VHAL_SWCSetdownSta_flg : BusSelector  OutputSignals=VHAL_SWCSetdownSta_flg
  slr_VHAL_SWCTripSta_flg : BusSelector  OutputSignals=VHAL_SWCTripSta_flg
  slr_VHAL_SWCUndefinedSta_flg : BusSelector  OutputSignals=VHAL_SWCUndefinedSta_flg
  slr_VHAL_SWCUpSta_flg : BusSelector  OutputSignals=VHAL_SWCUpSta_flg
  slr_VHAL_SWCVRSta_flg : BusSelector  OutputSignals=VHAL_SWCVRSta_flg
  slr_VHAL_SWCmodeSta_flg : BusSelector  OutputSignals=VHAL_SWCmodeSta_flg
  VINP_CSWDimSw_flg : Outport
  VINP_CSWFWasSwSta_enum : Outport  Port=2
  VINP_CSWFWipSwSta_enum : Outport  Port=3
  VINP_CSWPassSWSta_flg : Outport  Port=4
  VINP_CSWRWasSWSta_enum : Outport  Port=5
  VINP_CSWRWipIntSwSta_enum : Outport  Port=6
  VINP_CSWTurnSwSta_enum : Outport  Port=7
  VINP_FAPWL01LINResponseError_flg : Outport  Port=8
  VINP_LDrvMotorRelayError_flg : Outport  Port=9
  VINP_LDrvMotorRippleError_flg : Outport  Port=10
  VINP_LDrvValWdwOpened_pct : Outport  Port=11
  VINP_LDrvWdwPositionSts_enum : Outport  Port=12
  VINP_LPasMotorRelayError_flg : Outport  Port=13
  VINP_LPasMotorRippleError_flg : Outport  Port=14
  VINP_LPasValWdwOpened_pct : Outport  Port=15
  VINP_LPasWdwPositionSts_enum : Outport  Port=16
  VINP_LRLDMotorRelayError_flg : Outport  Port=17
  VINP_LRLDMotorRippleError_flg : Outport  Port=18
  VINP_LRLDValWdwOpened_pct : Outport  Port=19
  VINP_LRLDWdwPositionSts_enum : Outport  Port=20
  VINP_LRRDMotorRelayError_flg : Outport  Port=21
  VINP_LRRDMotorRippleError_flg : Outport  Port=22
  VINP_LRRDValWdwOpened_pct : Outport  Port=23
  VINP_LRRDWdwPositionSts_enum : Outport  Port=24
  VINP_RAPWL01LINResponseError_flg : Outport  Port=25
  VINP_RLSLampSta_flg : Outport  Port=26
  VINP_RLSRainSnrWiperCmd_enum : Outport  Port=27
  VINP_SWC2LADASSta_flg : Outport  Port=28
  VINP_SWC2LDriveModeSta_flg : Outport  Port=29
  VINP_SWC2LHomeSta_flg : Outport  Port=30
  VINP_SWC2LLeftSta_flg : Outport  Port=31
  VINP_SWC2LRegenUpSta_flg : Outport  Port=32
  VINP_SWC2LRightSta_flg : Outport  Port=33
  VINP_SWC2LScrollDownSta_flg : Outport  Port=34
  VINP_SWC2LScrollPressSta_flg : Outport  Port=35
  VINP_SWC2LScrollUpSta_flg : Outport  Port=36
  VINP_SWC2RCustomizeSta_flg : Outport  Port=37
  VINP_SWC2RLeftSta_flg : Outport  Port=38
  VINP_SWC2RPageSwitchSta_flg : Outport  Port=39
  VINP_SWC2RRegenDownSta_flg : Outport  Port=40
  VINP_SWC2RRightSta_flg : Outport  Port=41
  VINP_SWC2RScrollDownSta_flg : Outport  Port=42
  VINP_SWC2RScrollPressSta_flg : Outport  Port=43
  VINP_SWC2RScrollUpSta_flg : Outport  Port=44
  VINP_SWC2RVRSta_flg : Outport  Port=45
  VINP_SWCACCSta_flg : Outport  Port=46
  VINP_SWCCANCELSta_flg : Outport  Port=47
  VINP_SWCDistanceSta_flg : Outport  Port=48
  VINP_SWCDownSta_flg : Outport  Port=49
  VINP_SWCLKASta_flg : Outport  Port=50
  VINP_SWCLeftSta_flg : Outport  Port=51
  VINP_SWCRegenDown_flg : Outport  Port=52
  VINP_SWCRegenUp_flg : Outport  Port=53
  VINP_SWCResUpSta_flg : Outport  Port=54
  VINP_SWCRightSta_flg : Outport  Port=55
  VINP_SWCSetdownSta_flg : Outport  Port=56
  VINP_SWCTripSta_flg : Outport  Port=57
  VINP_SWCUndefinedSta_flg : Outport  Port=58
  VINP_SWCUpSta_flg : Outport  Port=59
  VINP_SWCVRSta_flg : Outport  Port=60
  VINP_SWCmodeSta_flg : Outport  Port=61
  wires:
  BHAL_outputs/1 -> [BHAL_outputs]
  inp_CanValid_bus/1 -> [inp_CanValid_bus]
  [BHAL_outputs] -> slr_VHAL_CSWDimSw_flg/1
  slr_VHAL_CSWDimSw_flg/1 -> CSWDimSw/1  "<VHAL_CSWDimSw_flg>"
  True_VHAL_CSWDimSw_flg/1 -> CSWDimSw/2
  [inp_CanValid_bus] -> slr1_1/1
  slr1_1/1 -> CSWDimSw/3  "<VINP_CANMsgValidzGWLINDr1_flg>"
  CSWDimSw/1 -> VINP_CSWDimSw_flg/1  "VINP_CSWDimSw_flg"
  CSWDimSw/2 -> Terminator_1/1
  [BHAL_outputs] -> slr_VHAL_CSWFWasSwSta_enum/1
  slr_VHAL_CSWFWasSwSta_enum/1 -> CSWFWasSwSta/1  "<VHAL_CSWFWasSwSta_enum>"
  True_VHAL_CSWFWasSwSta_enum/1 -> CSWFWasSwSta/2
  [inp_CanValid_bus] -> slr1_2/1
  slr1_2/1 -> CSWFWasSwSta/3  "<VINP_CANMsgValidzGWLINDr1_flg>"
  CSWFWasSwSta/1 -> VINP_CSWFWasSwSta_enum/1  "VINP_CSWFWasSwSta_enum"
  CSWFWasSwSta/2 -> Terminator_2/1
  [BHAL_outputs] -> slr_VHAL_CSWFWipSwSta_enum/1
  slr_VHAL_CSWFWipSwSta_enum/1 -> CSWFWipSwSta/1  "<VHAL_CSWFWipSwSta_enum>"
  True_VHAL_CSWFWipSwSta_enum/1 -> CSWFWipSwSta/2
  [inp_CanValid_bus] -> slr1_3/1
  slr1_3/1 -> CSWFWipSwSta/3  "<VINP_CANMsgValidzGWLINDr1_flg>"
  CSWFWipSwSta/1 -> VINP_CSWFWipSwSta_enum/1  "VINP_CSWFWipSwSta_enum"
  CSWFWipSwSta/2 -> Terminator_3/1
  [BHAL_outputs] -> slr_VHAL_CSWPassSWSta_flg/1
  slr_VHAL_CSWPassSWSta_flg/1 -> CSWPassSWSta/1  "<VHAL_CSWPassSWSta_flg>"
  True_VHAL_CSWPassSWSta_flg/1 -> CSWPassSWSta/2
  [inp_CanValid_bus] -> slr1_4/1
  slr1_4/1 -> CSWPassSWSta/3  "<VINP_CANMsgValidzGWLINDr1_flg>"
  CSWPassSWSta/1 -> VINP_CSWPassSWSta_flg/1  "VINP_CSWPassSWSta_flg"
  CSWPassSWSta/2 -> Terminator_4/1
  [BHAL_outputs] -> slr_VHAL_CSWRWasSWSta_enum/1
  slr_VHAL_CSWRWasSWSta_enum/1 -> CSWRWasSWSta/1  "<VHAL_CSWRWasSWSta_enum>"
  True_VHAL_CSWRWasSWSta_enum/1 -> CSWRWasSWSta/2
  [inp_CanValid_bus] -> slr1_5/1
  slr1_5/1 -> CSWRWasSWSta/3  "<VINP_CANMsgValidzGWLINDr1_flg>"
  CSWRWasSWSta/1 -> VINP_CSWRWasSWSta_enum/1  "VINP_CSWRWasSWSta_enum"
  CSWRWasSWSta/2 -> Terminator_5/1
  [BHAL_outputs] -> slr_VHAL_CSWRWipIntSwSta_enum/1
  slr_VHAL_CSWRWipIntSwSta_enum/1 -> CSWRWipIntSwSta/1  "<VHAL_CSWRWipIntSwSta_enum>"
  True_VHAL_CSWRWipIntSwSta_enum/1 -> CSWRWipIntSwSta/2
  [inp_CanValid_bus] -> slr1_6/1
  slr1_6/1 -> CSWRWipIntSwSta/3  "<VINP_CANMsgValidzGWLINDr1_flg>"
  CSWRWipIntSwSta/1 -> VINP_CSWRWipIntSwSta_enum/1  "VINP_CSWRWipIntSwSta_enum"
  CSWRWipIntSwSta/2 -> Terminator_6/1
  [BHAL_outputs] -> slr_VHAL_CSWTurnSwSta_enum/1
  slr_VHAL_CSWTurnSwSta_enum/1 -> CSWTurnSwSta/1  "<VHAL_CSWTurnSwSta_enum>"
  True_VHAL_CSWTurnSwSta_enum/1 -> CSWTurnSwSta/2
  [inp_CanValid_bus] -> slr1_7/1
  slr1_7/1 -> CSWTurnSwSta/3  "<VINP_CANMsgValidzGWLINDr1_flg>"
  CSWTurnSwSta/1 -> VINP_CSWTurnSwSta_enum/1  "VINP_CSWTurnSwSta_enum"
  CSWTurnSwSta/2 -> Terminator_7/1
  [BHAL_outputs] -> slr_VHAL_FAPWL01LINResponseError_flg/1
  slr_VHAL_FAPWL01LINResponseError_flg/1 -> FAPWL01LINResponseError/1  "<VHAL_FAPWL01LINResponseError_flg>"
  True_VHAL_FAPWL01LINResponseError_flg/1 -> FAPWL01LINResponseError/2
  [inp_CanValid_bus] -> slr1_8/1
  slr1_8/1 -> FAPWL01LINResponseError/3  "<VINP_CANMsgValidzGWLINDr1_flg>"
  FAPWL01LINResponseError/1 -> VINP_FAPWL01LINResponseError_flg/1  "VINP_FAPWL01LINResponseError_flg"
  FAPWL01LINResponseError/2 -> Terminator_8/1
  [BHAL_outputs] -> slr_VHAL_LDrvMotorRelayError_flg/1
  slr_VHAL_LDrvMotorRelayError_flg/1 -> LDrvMotorRelayError/1  "<VHAL_LDrvMotorRelayError_flg>"
  True_VHAL_LDrvMotorRelayError_flg/1 -> LDrvMotorRelayError/2
  [inp_CanValid_bus] -> slr1_9/1
  slr1_9/1 -> LDrvMotorRelayError/3  "<VINP_CANMsgValidzGWLINDr1_flg>"
  LDrvMotorRelayError/1 -> VINP_LDrvMotorRelayError_flg/1  "VINP_LDrvMotorRelayError_flg"
  LDrvMotorRelayError/2 -> Terminator_9/1
  [BHAL_outputs] -> slr_VHAL_LDrvMotorRippleError_flg/1
  slr_VHAL_LDrvMotorRippleError_flg/1 -> LDrvMotorRippleError/1  "<VHAL_LDrvMotorRippleError_flg>"
  True_VHAL_LDrvMotorRippleError_flg/1 -> LDrvMotorRippleError/2
  [inp_CanValid_bus] -> slr1_10/1
  slr1_10/1 -> LDrvMotorRippleError/3  "<VINP_CANMsgValidzGWLINDr1_flg>"
  LDrvMotorRippleError/1 -> VINP_LDrvMotorRippleError_flg/1  "VINP_LDrvMotorRippleError_flg"
  LDrvMotorRippleError/2 -> Terminator_10/1
  [BHAL_outputs] -> slr_VHAL_LDrvValWdwOpened_pct/1
  slr_VHAL_LDrvValWdwOpened_pct/1 -> LDrvValWdwOpened/1  "<VHAL_LDrvValWdwOpened_pct>"
  True_VHAL_LDrvValWdwOpened_pct/1 -> LDrvValWdwOpened/2
  [inp_CanValid_bus] -> slr1_11/1
  slr1_11/1 -> LDrvValWdwOpened/3  "<VINP_CANMsgValidzGWLINDr1_flg>"
  LDrvValWdwOpened/1 -> VINP_LDrvValWdwOpened_pct/1  "VINP_LDrvValWdwOpened_pct"
  LDrvValWdwOpened/2 -> Terminator_11/1
  [BHAL_outputs] -> slr_VHAL_LDrvWdwPositionSts_enum/1
  slr_VHAL_LDrvWdwPositionSts_enum/1 -> LDrvWdwPositionSts/1  "<VHAL_LDrvWdwPositionSts_enum>"
  True_VHAL_LDrvWdwPositionSts_enum/1 -> LDrvWdwPositionSts/2
  [inp_CanValid_bus] -> slr1_12/1
  slr1_12/1 -> LDrvWdwPositionSts/3  "<VINP_CANMsgValidzGWLINDr1_flg>"
  LDrvWdwPositionSts/1 -> VINP_LDrvWdwPositionSts_enum/1  "VINP_LDrvWdwPositionSts_enum"
  LDrvWdwPositionSts/2 -> Terminator_12/1
  [BHAL_outputs] -> slr_VHAL_LPasMotorRelayError_flg/1
  slr_VHAL_LPasMotorRelayError_flg/1 -> LPasMotorRelayError/1  "<VHAL_LPasMotorRelayError_flg>"
  True_VHAL_LPasMotorRelayError_flg/1 -> LPasMotorRelayError/2
  [inp_CanValid_bus] -> slr1_13/1
  slr1_13/1 -> LPasMotorRelayError/3  "<VINP_CANMsgValidzGWLINDr1_flg>"
  LPasMotorRelayError/1 -> VINP_LPasMotorRelayError_flg/1  "VINP_LPasMotorRelayError_flg"
  LPasMotorRelayError/2 -> Terminator_13/1
  [BHAL_outputs] -> slr_VHAL_LPasMotorRippleError_flg/1
  slr_VHAL_LPasMotorRippleError_flg/1 -> LPasMotorRippleError/1  "<VHAL_LPasMotorRippleError_flg>"
  True_VHAL_LPasMotorRippleError_flg/1 -> LPasMotorRippleError/2
  [inp_CanValid_bus] -> slr1_14/1
  slr1_14/1 -> LPasMotorRippleError/3  "<VINP_CANMsgValidzGWLINDr1_flg>"
  LPasMotorRippleError/1 -> VINP_LPasMotorRippleError_flg/1  "VINP_LPasMotorRippleError_flg"
  LPasMotorRippleError/2 -> Terminator_14/1
  [BHAL_outputs] -> slr_VHAL_LPasValWdwOpened_pct/1
  slr_VHAL_LPasValWdwOpened_pct/1 -> LPasValWdwOpened/1  "<VHAL_LPasValWdwOpened_pct>"
  True_VHAL_LPasValWdwOpened_pct/1 -> LPasValWdwOpened/2
  [inp_CanValid_bus] -> slr1_15/1
  slr1_15/1 -> LPasValWdwOpened/3  "<VINP_CANMsgValidzGWLINDr1_flg>"
  LPasValWdwOpened/1 -> VINP_LPasValWdwOpened_pct/1  "VINP_LPasValWdwOpened_pct"
  LPasValWdwOpened/2 -> Terminator_15/1
  [BHAL_outputs] -> slr_VHAL_LPasWdwPositionSts_enum/1
  slr_VHAL_LPasWdwPositionSts_enum/1 -> LPasWdwPositionSts/1  "<VHAL_LPasWdwPositionSts_enum>"
  True_VHAL_LPasWdwPositionSts_enum/1 -> LPasWdwPositionSts/2
  [inp_CanValid_bus] -> slr1_16/1
  slr1_16/1 -> LPasWdwPositionSts/3  "<VINP_CANMsgValidzGWLINDr1_flg>"
  LPasWdwPositionSts/1 -> VINP_LPasWdwPositionSts_enum/1  "VINP_LPasWdwPositionSts_enum"
  LPasWdwPositionSts/2 -> Terminator_16/1
  [BHAL_outputs] -> slr_VHAL_LRLDMotorRelayError_flg/1
  slr_VHAL_LRLDMotorRelayError_flg/1 -> LRLDMotorRelayError/1  "<VHAL_LRLDMotorRelayError_flg>"
  True_VHAL_LRLDMotorRelayError_flg/1 -> LRLDMotorRelayError/2
  [inp_CanValid_bus] -> slr1_17/1
  slr1_17/1 -> LRLDMotorRelayError/3  "<VINP_CANMsgValidzGWLINDr1_flg>"
  LRLDMotorRelayError/1 -> VINP_LRLDMotorRelayError_flg/1  "VINP_LRLDMotorRelayError_flg"
  LRLDMotorRelayError/2 -> Terminator_17/1
  [BHAL_outputs] -> slr_VHAL_LRLDMotorRippleError_flg/1
  slr_VHAL_LRLDMotorRippleError_flg/1 -> LRLDMotorRippleError/1  "<VHAL_LRLDMotorRippleError_flg>"
  True_VHAL_LRLDMotorRippleError_flg/1 -> LRLDMotorRippleError/2
  [inp_CanValid_bus] -> slr1_18/1
  slr1_18/1 -> LRLDMotorRippleError/3  "<VINP_CANMsgValidzGWLINDr1_flg>"
  LRLDMotorRippleError/1 -> VINP_LRLDMotorRippleError_flg/1  "VINP_LRLDMotorRippleError_flg"
  LRLDMotorRippleError/2 -> Terminator_18/1
  [BHAL_outputs] -> slr_VHAL_LRLDValWdwOpened_pct/1
  slr_VHAL_LRLDValWdwOpened_pct/1 -> LRLDValWdwOpened/1  "<VHAL_LRLDValWdwOpened_pct>"
  True_VHAL_LRLDValWdwOpened_pct/1 -> LRLDValWdwOpened/2
  [inp_CanValid_bus] -> slr1_19/1
  slr1_19/1 -> LRLDValWdwOpened/3  "<VINP_CANMsgValidzGWLINDr1_flg>"
  LRLDValWdwOpened/1 -> VINP_LRLDValWdwOpened_pct/1  "VINP_LRLDValWdwOpened_pct"
  LRLDValWdwOpened/2 -> Terminator_19/1
  [BHAL_outputs] -> slr_VHAL_LRLDWdwPositionSts_enum/1
  slr_VHAL_LRLDWdwPositionSts_enum/1 -> LRLDWdwPositionSts/1  "<VHAL_LRLDWdwPositionSts_enum>"
  True_VHAL_LRLDWdwPositionSts_enum/1 -> LRLDWdwPositionSts/2
  [inp_CanValid_bus] -> slr1_20/1
  slr1_20/1 -> LRLDWdwPositionSts/3  "<VINP_CANMsgValidzGWLINDr1_flg>"
  LRLDWdwPositionSts/1 -> VINP_LRLDWdwPositionSts_enum/1  "VINP_LRLDWdwPositionSts_enum"
  LRLDWdwPositionSts/2 -> Terminator_20/1
  [BHAL_outputs] -> slr_VHAL_LRRDMotorRelayError_flg/1
  slr_VHAL_LRRDMotorRelayError_flg/1 -> LRRDMotorRelayError/1  "<VHAL_LRRDMotorRelayError_flg>"
  True_VHAL_LRRDMotorRelayError_flg/1 -> LRRDMotorRelayError/2
  [inp_CanValid_bus] -> slr1_21/1
  slr1_21/1 -> LRRDMotorRelayError/3  "<VINP_CANMsgValidzGWLINDr1_flg>"
  LRRDMotorRelayError/1 -> VINP_LRRDMotorRelayError_flg/1  "VINP_LRRDMotorRelayError_flg"
  LRRDMotorRelayError/2 -> Terminator_21/1
  [BHAL_outputs] -> slr_VHAL_LRRDMotorRippleError_flg/1
  slr_VHAL_LRRDMotorRippleError_flg/1 -> LRRDMotorRippleError/1  "<VHAL_LRRDMotorRippleError_flg>"
  True_VHAL_LRRDMotorRippleError_flg/1 -> LRRDMotorRippleError/2
  [inp_CanValid_bus] -> slr1_22/1
  slr1_22/1 -> LRRDMotorRippleError/3  "<VINP_CANMsgValidzGWLINDr1_flg>"
  LRRDMotorRippleError/1 -> VINP_LRRDMotorRippleError_flg/1  "VINP_LRRDMotorRippleError_flg"
  LRRDMotorRippleError/2 -> Terminator_22/1
  [BHAL_outputs] -> slr_VHAL_LRRDValWdwOpened_pct/1
  slr_VHAL_LRRDValWdwOpened_pct/1 -> LRRDValWdwOpened/1  "<VHAL_LRRDValWdwOpened_pct>"
  True_VHAL_LRRDValWdwOpened_pct/1 -> LRRDValWdwOpened/2
  [inp_CanValid_bus] -> slr1_23/1
  slr1_23/1 -> LRRDValWdwOpened/3  "<VINP_CANMsgValidzGWLINDr1_flg>"
  LRRDValWdwOpened/1 -> VINP_LRRDValWdwOpened_pct/1  "VINP_LRRDValWdwOpened_pct"
  LRRDValWdwOpened/2 -> Terminator_23/1
  [BHAL_outputs] -> slr_VHAL_LRRDWdwPositionSts_enum/1
  slr_VHAL_LRRDWdwPositionSts_enum/1 -> LRRDWdwPositionSts/1  "<VHAL_LRRDWdwPositionSts_enum>"
  True_VHAL_LRRDWdwPositionSts_enum/1 -> LRRDWdwPositionSts/2
  [inp_CanValid_bus] -> slr1_24/1
  slr1_24/1 -> LRRDWdwPositionSts/3  "<VINP_CANMsgValidzGWLINDr1_flg>"
  LRRDWdwPositionSts/1 -> VINP_LRRDWdwPositionSts_enum/1  "VINP_LRRDWdwPositionSts_enum"
  LRRDWdwPositionSts/2 -> Terminator_24/1
  [BHAL_outputs] -> slr_VHAL_RAPWL01LINResponseError_flg/1
  slr_VHAL_RAPWL01LINResponseError_flg/1 -> RAPWL01LINResponseError/1  "<VHAL_RAPWL01LINResponseError_flg>"
  True_VHAL_RAPWL01LINResponseError_flg/1 -> RAPWL01LINResponseError/2
  [inp_CanValid_bus] -> slr1_25/1
  slr1_25/1 -> RAPWL01LINResponseError/3  "<VINP_CANMsgValidzGWLINDr1_flg>"
  RAPWL01LINResponseError/1 -> VINP_RAPWL01LINResponseError_flg/1  "VINP_RAPWL01LINResponseError_flg"
  RAPWL01LINResponseError/2 -> Terminator_25/1
  [BHAL_outputs] -> slr_VHAL_RLSLampSta_flg/1
  slr_VHAL_RLSLampSta_flg/1 -> RLSLampSta/1  "<VHAL_RLSLampSta_flg>"
  True_VHAL_RLSLampSta_flg/1 -> RLSLampSta/2
  [inp_CanValid_bus] -> slr1_26/1
  slr1_26/1 -> RLSLampSta/3  "<VINP_CANMsgValidzGWLINDr1_flg>"
  RLSLampSta/1 -> VINP_RLSLampSta_flg/1  "VINP_RLSLampSta_flg"
  RLSLampSta/2 -> Terminator_26/1
  [BHAL_outputs] -> slr_VHAL_RLSRainSnrWiperCmd_enum/1
  slr_VHAL_RLSRainSnrWiperCmd_enum/1 -> RLSRainSnrWiperCmd/1  "<VHAL_RLSRainSnrWiperCmd_enum>"
  True_VHAL_RLSRainSnrWiperCmd_enum/1 -> RLSRainSnrWiperCmd/2
  [inp_CanValid_bus] -> slr1_27/1
  slr1_27/1 -> RLSRainSnrWiperCmd/3  "<VINP_CANMsgValidzGWLINDr1_flg>"
  RLSRainSnrWiperCmd/1 -> VINP_RLSRainSnrWiperCmd_enum/1  "VINP_RLSRainSnrWiperCmd_enum"
  RLSRainSnrWiperCmd/2 -> Terminator_27/1
  [BHAL_outputs] -> slr_VHAL_SWC2LADASSta_flg/1
  slr_VHAL_SWC2LADASSta_flg/1 -> SWC2LADASSta/1  "<VHAL_SWC2LADASSta_flg>"
  True_VHAL_SWC2LADASSta_flg/1 -> SWC2LADASSta/2
  [inp_CanValid_bus] -> slr1_28/1
  slr1_28/1 -> SWC2LADASSta/3  "<VINP_CANMsgValidzGWLINDr1_flg>"
  SWC2LADASSta/1 -> VINP_SWC2LADASSta_flg/1  "VINP_SWC2LADASSta_flg"
  SWC2LADASSta/2 -> Terminator_28/1
  [BHAL_outputs] -> slr_VHAL_SWC2LDriveModeSta_flg/1
  slr_VHAL_SWC2LDriveModeSta_flg/1 -> SWC2LDriveModeSta/1  "<VHAL_SWC2LDriveModeSta_flg>"
  True_VHAL_SWC2LDriveModeSta_flg/1 -> SWC2LDriveModeSta/2
  [inp_CanValid_bus] -> slr1_29/1
  slr1_29/1 -> SWC2LDriveModeSta/3  "<VINP_CANMsgValidzGWLINDr1_flg>"
  SWC2LDriveModeSta/1 -> VINP_SWC2LDriveModeSta_flg/1  "VINP_SWC2LDriveModeSta_flg"
  SWC2LDriveModeSta/2 -> Terminator_29/1
  [BHAL_outputs] -> slr_VHAL_SWC2LHomeSta_flg/1
  slr_VHAL_SWC2LHomeSta_flg/1 -> SWC2LHomeSta/1  "<VHAL_SWC2LHomeSta_flg>"
  True_VHAL_SWC2LHomeSta_flg/1 -> SWC2LHomeSta/2
  [inp_CanValid_bus] -> slr1_30/1
  slr1_30/1 -> SWC2LHomeSta/3  "<VINP_CANMsgValidzGWLINDr1_flg>"
  SWC2LHomeSta/1 -> VINP_SWC2LHomeSta_flg/1  "VINP_SWC2LHomeSta_flg"
  SWC2LHomeSta/2 -> Terminator_30/1
  [BHAL_outputs] -> slr_VHAL_SWC2LLeftSta_flg/1
  slr_VHAL_SWC2LLeftSta_flg/1 -> SWC2LLeftSta/1  "<VHAL_SWC2LLeftSta_flg>"
  True_VHAL_SWC2LLeftSta_flg/1 -> SWC2LLeftSta/2
  [inp_CanValid_bus] -> slr1_31/1
  slr1_31/1 -> SWC2LLeftSta/3  "<VINP_CANMsgValidzGWLINDr1_flg>"
  SWC2LLeftSta/1 -> VINP_SWC2LLeftSta_flg/1  "VINP_SWC2LLeftSta_flg"
  SWC2LLeftSta/2 -> Terminator_31/1
  [BHAL_outputs] -> slr_VHAL_SWC2LRegenUpSta_flg/1
  slr_VHAL_SWC2LRegenUpSta_flg/1 -> SWC2LRegenUpSta/1  "<VHAL_SWC2LRegenUpSta_flg>"
  True_VHAL_SWC2LRegenUpSta_flg/1 -> SWC2LRegenUpSta/2
  [inp_CanValid_bus] -> slr1_32/1
  slr1_32/1 -> SWC2LRegenUpSta/3  "<VINP_CANMsgValidzGWLINDr1_flg>"
  SWC2LRegenUpSta/1 -> VINP_SWC2LRegenUpSta_flg/1  "VINP_SWC2LRegenUpSta_flg"
  SWC2LRegenUpSta/2 -> Terminator_32/1
  [BHAL_outputs] -> slr_VHAL_SWC2LRightSta_flg/1
  slr_VHAL_SWC2LRightSta_flg/1 -> SWC2LRightSta/1  "<VHAL_SWC2LRightSta_flg>"
  True_VHAL_SWC2LRightSta_flg/1 -> SWC2LRightSta/2
  [inp_CanValid_bus] -> slr1_33/1
  slr1_33/1 -> SWC2LRightSta/3  "<VINP_CANMsgValidzGWLINDr1_flg>"
  SWC2LRightSta/1 -> VINP_SWC2LRightSta_flg/1  "VINP_SWC2LRightSta_flg"
  SWC2LRightSta/2 -> Terminator_33/1
  [BHAL_outputs] -> slr_VHAL_SWC2LScrollDownSta_flg/1
  slr_VHAL_SWC2LScrollDownSta_flg/1 -> SWC2LScrollDownSta/1  "<VHAL_SWC2LScrollDownSta_flg>"
  True_VHAL_SWC2LScrollDownSta_flg/1 -> SWC2LScrollDownSta/2
  [inp_CanValid_bus] -> slr1_34/1
  slr1_34/1 -> SWC2LScrollDownSta/3  "<VINP_CANMsgValidzGWLINDr1_flg>"
  SWC2LScrollDownSta/1 -> VINP_SWC2LScrollDownSta_flg/1  "VINP_SWC2LScrollDownSta_flg"
  SWC2LScrollDownSta/2 -> Terminator_34/1
  [BHAL_outputs] -> slr_VHAL_SWC2LScrollPressSta_flg/1
  slr_VHAL_SWC2LScrollPressSta_flg/1 -> SWC2LScrollPressSta/1  "<VHAL_SWC2LScrollPressSta_flg>"
  True_VHAL_SWC2LScrollPressSta_flg/1 -> SWC2LScrollPressSta/2
  [inp_CanValid_bus] -> slr1_35/1
  slr1_35/1 -> SWC2LScrollPressSta/3  "<VINP_CANMsgValidzGWLINDr1_flg>"
  SWC2LScrollPressSta/1 -> VINP_SWC2LScrollPressSta_flg/1  "VINP_SWC2LScrollPressSta_flg"
  SWC2LScrollPressSta/2 -> Terminator_35/1
  [BHAL_outputs] -> slr_VHAL_SWC2LScrollUpSta_flg/1
  slr_VHAL_SWC2LScrollUpSta_flg/1 -> SWC2LScrollUpSta/1  "<VHAL_SWC2LScrollUpSta_flg>"
  True_VHAL_SWC2LScrollUpSta_flg/1 -> SWC2LScrollUpSta/2
  [inp_CanValid_bus] -> slr1_36/1
  slr1_36/1 -> SWC2LScrollUpSta/3  "<VINP_CANMsgValidzGWLINDr1_flg>"
  SWC2LScrollUpSta/1 -> VINP_SWC2LScrollUpSta_flg/1  "VINP_SWC2LScrollUpSta_flg"
  SWC2LScrollUpSta/2 -> Terminator_36/1
  [BHAL_outputs] -> slr_VHAL_SWC2RCustomizeSta_flg/1
  slr_VHAL_SWC2RCustomizeSta_flg/1 -> SWC2RCustomizeSta/1  "<VHAL_SWC2RCustomizeSta_flg>"
  True_VHAL_SWC2RCustomizeSta_flg/1 -> SWC2RCustomizeSta/2
  [inp_CanValid_bus] -> slr1_37/1
  slr1_37/1 -> SWC2RCustomizeSta/3  "<VINP_CANMsgValidzGWLINDr1_flg>"
  SWC2RCustomizeSta/1 -> VINP_SWC2RCustomizeSta_flg/1  "VINP_SWC2RCustomizeSta_flg"
  SWC2RCustomizeSta/2 -> Terminator_37/1
  [BHAL_outputs] -> slr_VHAL_SWC2RLeftSta_flg/1
  slr_VHAL_SWC2RLeftSta_flg/1 -> SWC2RLeftSta/1  "<VHAL_SWC2RLeftSta_flg>"
  True_VHAL_SWC2RLeftSta_flg/1 -> SWC2RLeftSta/2
  [inp_CanValid_bus] -> slr1_38/1
  slr1_38/1 -> SWC2RLeftSta/3  "<VINP_CANMsgValidzGWLINDr1_flg>"
  SWC2RLeftSta/1 -> VINP_SWC2RLeftSta_flg/1  "VINP_SWC2RLeftSta_flg"
  SWC2RLeftSta/2 -> Terminator_38/1
  [BHAL_outputs] -> slr_VHAL_SWC2RPageSwitchSta_flg/1
  slr_VHAL_SWC2RPageSwitchSta_flg/1 -> SWC2RPageSwitchSta/1  "<VHAL_SWC2RPageSwitchSta_flg>"
  True_VHAL_SWC2RPageSwitchSta_flg/1 -> SWC2RPageSwitchSta/2
  [inp_CanValid_bus] -> slr1_39/1
  slr1_39/1 -> SWC2RPageSwitchSta/3  "<VINP_CANMsgValidzGWLINDr1_flg>"
  SWC2RPageSwitchSta/1 -> VINP_SWC2RPageSwitchSta_flg/1  "VINP_SWC2RPageSwitchSta_flg"
  SWC2RPageSwitchSta/2 -> Terminator_39/1
  [BHAL_outputs] -> slr_VHAL_SWC2RRegenDownSta_flg/1
  slr_VHAL_SWC2RRegenDownSta_flg/1 -> SWC2RRegenDownSta/1  "<VHAL_SWC2RRegenDownSta_flg>"
  True_VHAL_SWC2RRegenDownSta_flg/1 -> SWC2RRegenDownSta/2
  [inp_CanValid_bus] -> slr1_40/1
  slr1_40/1 -> SWC2RRegenDownSta/3  "<VINP_CANMsgValidzGWLINDr1_flg>"
  SWC2RRegenDownSta/1 -> VINP_SWC2RRegenDownSta_flg/1  "VINP_SWC2RRegenDownSta_flg"
  SWC2RRegenDownSta/2 -> Terminator_40/1
  [BHAL_outputs] -> slr_VHAL_SWC2RRightSta_flg/1
  slr_VHAL_SWC2RRightSta_flg/1 -> SWC2RRightSta/1  "<VHAL_SWC2RRightSta_flg>"
  True_VHAL_SWC2RRightSta_flg/1 -> SWC2RRightSta/2
  [inp_CanValid_bus] -> slr1_41/1
  slr1_41/1 -> SWC2RRightSta/3  "<VINP_CANMsgValidzGWLINDr1_flg>"
  SWC2RRightSta/1 -> VINP_SWC2RRightSta_flg/1  "VINP_SWC2RRightSta_flg"
  SWC2RRightSta/2 -> Terminator_41/1
  [BHAL_outputs] -> slr_VHAL_SWC2RScrollDownSta_flg/1
  slr_VHAL_SWC2RScrollDownSta_flg/1 -> SWC2RScrollDownSta/1  "<VHAL_SWC2RScrollDownSta_flg>"
  True_VHAL_SWC2RScrollDownSta_flg/1 -> SWC2RScrollDownSta/2
  [inp_CanValid_bus] -> slr1_42/1
  slr1_42/1 -> SWC2RScrollDownSta/3  "<VINP_CANMsgValidzGWLINDr1_flg>"
  SWC2RScrollDownSta/1 -> VINP_SWC2RScrollDownSta_flg/1  "VINP_SWC2RScrollDownSta_flg"
  SWC2RScrollDownSta/2 -> Terminator_42/1
  [BHAL_outputs] -> slr_VHAL_SWC2RScrollPressSta_flg/1
  slr_VHAL_SWC2RScrollPressSta_flg/1 -> SWC2RScrollPressSta/1  "<VHAL_SWC2RScrollPressSta_flg>"
  True_VHAL_SWC2RScrollPressSta_flg/1 -> SWC2RScrollPressSta/2
  [inp_CanValid_bus] -> slr1_43/1
  slr1_43/1 -> SWC2RScrollPressSta/3  "<VINP_CANMsgValidzGWLINDr1_flg>"
  SWC2RScrollPressSta/1 -> VINP_SWC2RScrollPressSta_flg/1  "VINP_SWC2RScrollPressSta_flg"
  SWC2RScrollPressSta/2 -> Terminator_43/1
  [BHAL_outputs] -> slr_VHAL_SWC2RScrollUpSta_flg/1
  slr_VHAL_SWC2RScrollUpSta_flg/1 -> SWC2RScrollUpSta/1  "<VHAL_SWC2RScrollUpSta_flg>"
  True_VHAL_SWC2RScrollUpSta_flg/1 -> SWC2RScrollUpSta/2
  [inp_CanValid_bus] -> slr1_44/1
  slr1_44/1 -> SWC2RScrollUpSta/3  "<VINP_CANMsgValidzGWLINDr1_flg>"
  SWC2RScrollUpSta/1 -> VINP_SWC2RScrollUpSta_flg/1  "VINP_SWC2RScrollUpSta_flg"
  SWC2RScrollUpSta/2 -> Terminator_44/1
  [BHAL_outputs] -> slr_VHAL_SWC2RVRSta_flg/1
  slr_VHAL_SWC2RVRSta_flg/1 -> SWC2RVRSta/1  "<VHAL_SWC2RVRSta_flg>"
  True_VHAL_SWC2RVRSta_flg/1 -> SWC2RVRSta/2
  [inp_CanValid_bus] -> slr1_45/1
  slr1_45/1 -> SWC2RVRSta/3  "<VINP_CANMsgValidzGWLINDr1_flg>"
  SWC2RVRSta/1 -> VINP_SWC2RVRSta_flg/1  "VINP_SWC2RVRSta_flg"
  SWC2RVRSta/2 -> Terminator_45/1
  [BHAL_outputs] -> slr_VHAL_SWCACCSta_flg/1
  slr_VHAL_SWCACCSta_flg/1 -> SWCACCSta/1  "<VHAL_SWCACCSta_flg>"
  True_VHAL_SWCACCSta_flg/1 -> SWCACCSta/2
  [inp_CanValid_bus] -> slr1_46/1
  slr1_46/1 -> SWCACCSta/3  "<VINP_CANMsgValidzGWLINDr1_flg>"
  SWCACCSta/1 -> VINP_SWCACCSta_flg/1  "VINP_SWCACCSta_flg"
  SWCACCSta/2 -> Terminator_46/1
  [BHAL_outputs] -> slr_VHAL_SWCCANCELSta_flg/1
  slr_VHAL_SWCCANCELSta_flg/1 -> SWCCANCELSta/1  "<VHAL_SWCCANCELSta_flg>"
  True_VHAL_SWCCANCELSta_flg/1 -> SWCCANCELSta/2
  [inp_CanValid_bus] -> slr1_47/1
  slr1_47/1 -> SWCCANCELSta/3  "<VINP_CANMsgValidzGWLINDr1_flg>"
  SWCCANCELSta/1 -> VINP_SWCCANCELSta_flg/1  "VINP_SWCCANCELSta_flg"
  SWCCANCELSta/2 -> Terminator_47/1
  [BHAL_outputs] -> slr_VHAL_SWCDistanceSta_flg/1
  slr_VHAL_SWCDistanceSta_flg/1 -> SWCDistanceSta/1  "<VHAL_SWCDistanceSta_flg>"
  True_VHAL_SWCDistanceSta_flg/1 -> SWCDistanceSta/2
  [inp_CanValid_bus] -> slr1_48/1
  slr1_48/1 -> SWCDistanceSta/3  "<VINP_CANMsgValidzGWLINDr1_flg>"
  SWCDistanceSta/1 -> VINP_SWCDistanceSta_flg/1  "VINP_SWCDistanceSta_flg"
  SWCDistanceSta/2 -> Terminator_48/1
  [BHAL_outputs] -> slr_VHAL_SWCDownSta_flg/1
  slr_VHAL_SWCDownSta_flg/1 -> SWCDownSta/1  "<VHAL_SWCDownSta_flg>"
  True_VHAL_SWCDownSta_flg/1 -> SWCDownSta/2
  [inp_CanValid_bus] -> slr1_49/1
  slr1_49/1 -> SWCDownSta/3  "<VINP_CANMsgValidzGWLINDr1_flg>"
  SWCDownSta/1 -> VINP_SWCDownSta_flg/1  "VINP_SWCDownSta_flg"
  SWCDownSta/2 -> Terminator_49/1
  [BHAL_outputs] -> slr_VHAL_SWCLKASta_flg/1
  slr_VHAL_SWCLKASta_flg/1 -> SWCLKASta/1  "<VHAL_SWCLKASta_flg>"
  True_VHAL_SWCLKASta_flg/1 -> SWCLKASta/2
  [inp_CanValid_bus] -> slr1_50/1
  slr1_50/1 -> SWCLKASta/3  "<VINP_CANMsgValidzGWLINDr1_flg>"
  SWCLKASta/1 -> VINP_SWCLKASta_flg/1  "VINP_SWCLKASta_flg"
  SWCLKASta/2 -> Terminator_50/1
  [BHAL_outputs] -> slr_VHAL_SWCLeftSta_flg/1
  slr_VHAL_SWCLeftSta_flg/1 -> SWCLeftSta/1  "<VHAL_SWCLeftSta_flg>"
  True_VHAL_SWCLeftSta_flg/1 -> SWCLeftSta/2
  [inp_CanValid_bus] -> slr1_51/1
  slr1_51/1 -> SWCLeftSta/3  "<VINP_CANMsgValidzGWLINDr1_flg>"
  SWCLeftSta/1 -> VINP_SWCLeftSta_flg/1  "VINP_SWCLeftSta_flg"
  SWCLeftSta/2 -> Terminator_51/1
  [BHAL_outputs] -> slr_VHAL_SWCRegenDown_flg/1
  slr_VHAL_SWCRegenDown_flg/1 -> SWCRegenDown/1  "<VHAL_SWCRegenDown_flg>"
  True_VHAL_SWCRegenDown_flg/1 -> SWCRegenDown/2
  [inp_CanValid_bus] -> slr1_52/1
  slr1_52/1 -> SWCRegenDown/3  "<VINP_CANMsgValidzGWLINDr1_flg>"
  SWCRegenDown/1 -> VINP_SWCRegenDown_flg/1  "VINP_SWCRegenDown_flg"
  SWCRegenDown/2 -> Terminator_52/1
  [BHAL_outputs] -> slr_VHAL_SWCRegenUp_flg/1
  slr_VHAL_SWCRegenUp_flg/1 -> SWCRegenUp/1  "<VHAL_SWCRegenUp_flg>"
  True_VHAL_SWCRegenUp_flg/1 -> SWCRegenUp/2
  [inp_CanValid_bus] -> slr1_53/1
  slr1_53/1 -> SWCRegenUp/3  "<VINP_CANMsgValidzGWLINDr1_flg>"
  SWCRegenUp/1 -> VINP_SWCRegenUp_flg/1  "VINP_SWCRegenUp_flg"
  SWCRegenUp/2 -> Terminator_53/1
  [BHAL_outputs] -> slr_VHAL_SWCResUpSta_flg/1
  slr_VHAL_SWCResUpSta_flg/1 -> SWCResUpSta/1  "<VHAL_SWCResUpSta_flg>"
  True_VHAL_SWCResUpSta_flg/1 -> SWCResUpSta/2
  [inp_CanValid_bus] -> slr1_54/1
  slr1_54/1 -> SWCResUpSta/3  "<VINP_CANMsgValidzGWLINDr1_flg>"
  SWCResUpSta/1 -> VINP_SWCResUpSta_flg/1  "VINP_SWCResUpSta_flg"
  SWCResUpSta/2 -> Terminator_54/1
  [BHAL_outputs] -> slr_VHAL_SWCRightSta_flg/1
  slr_VHAL_SWCRightSta_flg/1 -> SWCRightSta/1  "<VHAL_SWCRightSta_flg>"
  True_VHAL_SWCRightSta_flg/1 -> SWCRightSta/2
  [inp_CanValid_bus] -> slr1_55/1
  slr1_55/1 -> SWCRightSta/3  "<VINP_CANMsgValidzGWLINDr1_flg>"
  SWCRightSta/1 -> VINP_SWCRightSta_flg/1  "VINP_SWCRightSta_flg"
  SWCRightSta/2 -> Terminator_55/1
  [BHAL_outputs] -> slr_VHAL_SWCSetdownSta_flg/1
  slr_VHAL_SWCSetdownSta_flg/1 -> SWCSetdownSta/1  "<VHAL_SWCSetdownSta_flg>"
  True_VHAL_SWCSetdownSta_flg/1 -> SWCSetdownSta/2
  [inp_CanValid_bus] -> slr1_56/1
  slr1_56/1 -> SWCSetdownSta/3  "<VINP_CANMsgValidzGWLINDr1_flg>"
  SWCSetdownSta/1 -> VINP_SWCSetdownSta_flg/1  "VINP_SWCSetdownSta_flg"
  SWCSetdownSta/2 -> Terminator_56/1
  [BHAL_outputs] -> slr_VHAL_SWCTripSta_flg/1
  slr_VHAL_SWCTripSta_flg/1 -> SWCTripSta/1  "<VHAL_SWCTripSta_flg>"
  True_VHAL_SWCTripSta_flg/1 -> SWCTripSta/2
  [inp_CanValid_bus] -> slr1_57/1
  slr1_57/1 -> SWCTripSta/3  "<VINP_CANMsgValidzGWLINDr1_flg>"
  SWCTripSta/1 -> VINP_SWCTripSta_flg/1  "VINP_SWCTripSta_flg"
  SWCTripSta/2 -> Terminator_57/1
  [BHAL_outputs] -> slr_VHAL_SWCUndefinedSta_flg/1
  slr_VHAL_SWCUndefinedSta_flg/1 -> SWCUndefinedSta/1  "<VHAL_SWCUndefinedSta_flg>"
  True_VHAL_SWCUndefinedSta_flg/1 -> SWCUndefinedSta/2
  [inp_CanValid_bus] -> slr1_58/1
  slr1_58/1 -> SWCUndefinedSta/3  "<VINP_CANMsgValidzGWLINDr1_flg>"
  SWCUndefinedSta/1 -> VINP_SWCUndefinedSta_flg/1  "VINP_SWCUndefinedSta_flg"
  SWCUndefinedSta/2 -> Terminator_58/1
  [BHAL_outputs] -> slr_VHAL_SWCUpSta_flg/1
  slr_VHAL_SWCUpSta_flg/1 -> SWCUpSta/1  "<VHAL_SWCUpSta_flg>"
  True_VHAL_SWCUpSta_flg/1 -> SWCUpSta/2
  [inp_CanValid_bus] -> slr1_59/1
  slr1_59/1 -> SWCUpSta/3  "<VINP_CANMsgValidzGWLINDr1_flg>"
  SWCUpSta/1 -> VINP_SWCUpSta_flg/1  "VINP_SWCUpSta_flg"
  SWCUpSta/2 -> Terminator_59/1
  [BHAL_outputs] -> slr_VHAL_SWCVRSta_flg/1
  slr_VHAL_SWCVRSta_flg/1 -> SWCVRSta/1  "<VHAL_SWCVRSta_flg>"
  True_VHAL_SWCVRSta_flg/1 -> SWCVRSta/2
  [inp_CanValid_bus] -> slr1_60/1
  slr1_60/1 -> SWCVRSta/3  "<VINP_CANMsgValidzGWLINDr1_flg>"
  SWCVRSta/1 -> VINP_SWCVRSta_flg/1  "VINP_SWCVRSta_flg"
  SWCVRSta/2 -> Terminator_60/1
  [BHAL_outputs] -> slr_VHAL_SWCmodeSta_flg/1
  slr_VHAL_SWCmodeSta_flg/1 -> SWCmodeSta/1  "<VHAL_SWCmodeSta_flg>"
  True_VHAL_SWCmodeSta_flg/1 -> SWCmodeSta/2
  [inp_CanValid_bus] -> slr1_61/1
  slr1_61/1 -> SWCmodeSta/3  "<VINP_CANMsgValidzGWLINDr1_flg>"
  SWCmodeSta/1 -> VINP_SWCmodeSta_flg/1  "VINP_SWCmodeSta_flg"
  SWCmodeSta/2 -> Terminator_61/1
